simulink model "Bicycle_LKS"  (R2017a)
settings: Solver=ode45  StartTime=0.0  StopTime=20  FixedStep=1/120  MaxStep=1/120  RelTol=1e-3  EnableMultiTasking=on
InitFcn:
  | % Load matfile %
  | load('Matrix.mat')
  | load('PathData.mat')
  | 
  | % 차량의 초기 위치 및 속도 설정 %
  | X0 = 25;            % 초기 X좌표 [m]
  | Y0 = 0.00138;       % 초기 Y좌표 [m]
  | psi0 = -0.6*pi/180; % 초기 각도 [rad]
  | Vx0 = 100;          % 초기 속도 [km/h]
  | tf = 30;            % 시뮬레이션 시간 [s]
  | 
  | % % 제어기 설정 %
  | Q1 = 5;        % Lateral Offset 의 가중치
  | Q2 = 30;        % Drift Angle의 가중치
  | R =  250;       % Steering Angle의 가중치
  | PL = [-50-50i,-50+50i,-30,-20]; % Observer 극점
  | 
  | [K,L] = sfGain(Q1,Q2,R,PL);
model workspace (MAT data in the model file):
  Cf = 53220
  Cr = 39017
  Fy_Angle = [-20; -16; -14; -12; -10; -9.5; -9; -8.5; -8; -7.5; -7; -6.5; -6; -5.5; -5; -4.5; -4; -3.5; -3; -2.5; -2; -1.5; -1; -0.5; 0; 0.5; 1; 1.5; 2; 2.5; 3; 3.5; 4; 4.5; 5; 5.5; 6; 6.5; 7; 7.5; 8; 8.5; 9; 9.5; 10; 12; 14; 16; 18; 20]
  Fy_Data = [-1523.64 -1531.91 -1546.58 -1574.53 -1631.62 -1653.27 -1678.67 -1707.8 -1740.18 -1775.12 -1810.95 -1845.3 ... (250 elements, 50x5)]
  Fy_W = [1725 3500 6100 6950 9005]
  GearRatio = 17.25
  Izz = 4192
  P = [2.59634065709e-08 -1.77089434361e-05 0.0015503820009 -0.0564733379764 0.710785401626]
  lf = 1.11
  lr = 1.6662
  m = 1530
values from neighbouring files (symbols this model uses):
  K = lqr(A,B,Q,R)    [sfGain.m]
  L = place(A',C',PL)    [sfGain.m]
undefined symbols (not defined in the file or in its folder): A, B
libraries: simulink x1
settings Model: Creator=Park  LastModifiedBy=edward
settings DataIOCC: SaveFormat=Array  SignalLoggingSaveFormat=ModelDataLogs
settings OptimizationCC: ExpressionDepthLimit=2147483647  LifeSpan=inf
settings DebuggingCC: UnderspecifiedInitializationDetection=Classic  MergeDetectMultiDrivingBlocksExec=none  SolverPrmCheckMsg=warning  MultiTaskDSMMsg=warning  MultiTaskCondExecSysMsg=none  FcnCallInpInsideContextMsg=warning  StateNameClashWarn=warning  SFUnexpectedBacktrackingDiag=warning  SFNoUnconditionalDefaultTransitionDiag=warning  SFExecutionAtInitializationDiag=none
settings HardwareCC: ProdBitPerPointer=32  ProdBitPerSizeT=32  ProdBitPerPtrDiffT=32  ProdLargestAtomicFloat=None  ProdIntDivRoundTo=Undefined  ProdEndianess=Unspecified  ProdWordSize=32  ProdHWDeviceType=32-bit Generic
settings ModelReferenceCC: PropagateSignalLabelsOutOfModel=off
settings GRTTargetCC: TargetLangStandard=C89/C90 (ANSI)  GeneratePreprocessorConditionals=Disable all  CombineOutputUpdateFcns=off  GRTInterface=on
settings ConfigComp: CovMetricSettings=dw  CovHtmlReporting=on  CovSaveCumulativeToWorkspaceVar=on  CovSaveSingleToWorkspaceVar=on  CovExternalEMLEnable=off

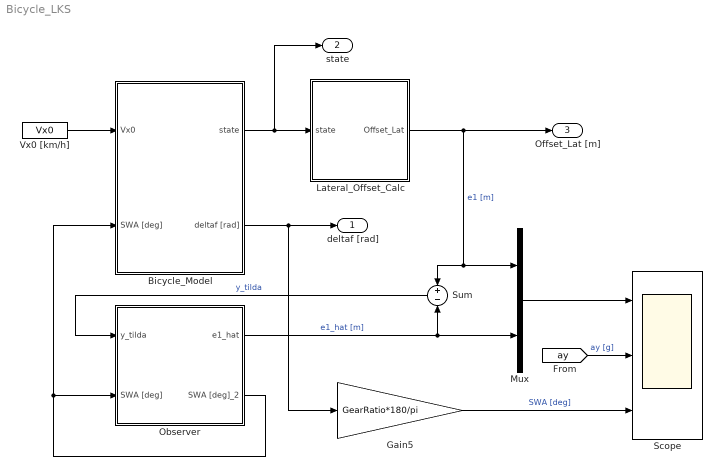
== system Bicycle_LKS ==
  Bicycle_Model : Subsystem
  Gain5 : Gain  Gain=GearRatio*180/pi
  Lateral_Offset_Calc : Subsystem  TreatAsAtomicUnit=on  SystemSampleTime=1/120
  Mux : Mux  Inputs=2
  Observer : Subsystem
  Scope : Scope  NumInputPorts=3
  Sum : Sum  Inputs=+-
  Vx0 [km/h] : Constant  Value=Vx0
  deltaf [rad] : Outport
  state : Outport  Port=2
  Offset_Lat [m] : Outport  Port=3
  wires:
  Bicycle_Model/1(state) -> Lateral_Offset_Calc/1(state), state/1
  Lateral_Offset_Calc/1(Offset_Lat) -> Offset_Lat [m]/1, Sum/1, Mux/1  "e1 [m]"
  Observer/1(e1_hat) -> Sum/2, Mux/2  "e1_hat [m]"
  Vx0 [km/h]/1 -> Bicycle_Model/1(Vx0)
  Sum/1 -> Observer/1(y_tilda)  "y_tilda"
  Mux/1 -> Scope/1
  [ay] -> Scope/2  "ay [g]"
  Bicycle_Model/2(deltaf [rad]) -> Gain5/1, deltaf [rad]/1
  Gain5/1 -> Scope/3  "SWA [deg]"
  Observer/2(SWA [deg]_2) -> Observer/2(SWA [deg]), Bicycle_Model/2(SWA [deg])

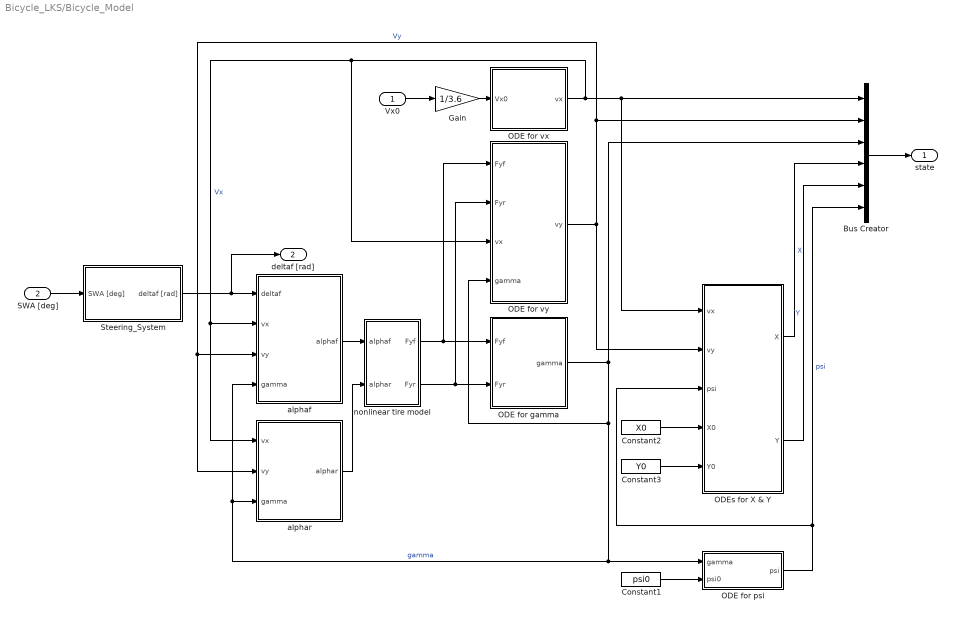
== system Bicycle_LKS/Bicycle_Model ==
  Vx0 : Inport
  SWA [deg] : Inport  Port=2
  Bus Creator : BusCreator  Inputs=6
  Constant1 : Constant  Value=psi0
  Constant2 : Constant  Value=X0
  Constant3 : Constant  Value=Y0
  Gain : Gain  Gain=1/3.6
  ODE for gamma : Subsystem
  ODE for psi : Subsystem
  ODE for vx : Subsystem
  ODE for vy : Subsystem
  ODEs for X & Y : Subsystem
  Steering_System : Subsystem
  alphaf : Subsystem
  alphar : Subsystem
  nonlinear tire model : Subsystem
  state : Outport
  deltaf [rad] : Outport  Port=2
  wires:
  alphaf/1(alphaf) -> nonlinear tire model/1(alphaf)
  alphar/1(alphar) -> nonlinear tire model/2(alphar)
  nonlinear tire model/1(Fyf) -> ODE for gamma/1(Fyf), ODE for vy/1(Fyf)
  nonlinear tire model/2(Fyr) -> ODE for gamma/2(Fyr), ODE for vy/2(Fyr)
  ODE for gamma/1(gamma) -> ODE for vy/4(gamma), alphar/3(gamma), alphaf/4(gamma), ODE for psi/1(gamma), Bus Creator/3  "gamma"
  ODE for vy/1(vy) -> Bus Creator/2, alphaf/3(vy), alphar/2(vy), ODEs for X & Y/2(vy)  "Vy"
  Bus Creator/1 -> state/1
  ODE for vx/1(vx) -> Bus Creator/1, ODEs for X & Y/1(vx), alphaf/2(vx), alphar/1(vx), ODE for vy/3(vx)  "Vx"
  Vx0/1 -> Gain/1
  Constant1/1 -> ODE for psi/2(psi0)
  Gain/1 -> ODE for vx/1(Vx0)
  SWA [deg]/1 -> Steering_System/1(SWA [deg])
  Steering_System/1(deltaf [rad]) -> deltaf [rad]/1, alphaf/1(deltaf)
  Constant2/1 -> ODEs for X & Y/4(X0)
  Constant3/1 -> ODEs for X & Y/5(Y0)
  ODE for psi/1(psi) -> Bus Creator/6, ODEs for X & Y/3(psi)  "psi"
  ODEs for X & Y/1(X) -> Bus Creator/4  "X"
  ODEs for X & Y/2(Y) -> Bus Creator/5  "Y"

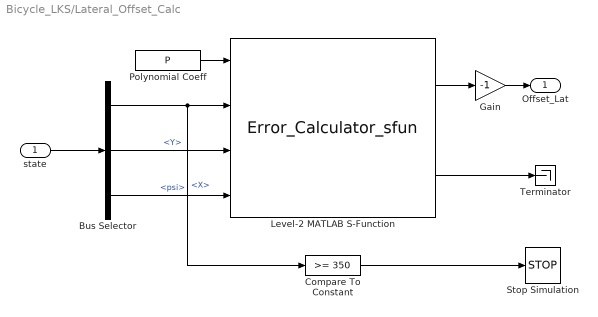
== system Bicycle_LKS/Lateral_Offset_Calc ==
  state : Inport
  Bus Selector : BusSelector  OutputSignals=X,Y,psi
  Compare To Constant : simulink/Logic and Bit Operations/Compare To Constant  relop=>=  const=350  OutDataTypeStr=boolean
  Gain : Gain  Gain=-1
  Level-2 MATLAB S-Function : M-S-Function  FunctionName=Error_Calculator_sfun
  Polynomial Coeff : Constant  Value=P
  Stop Simulation : Stop
  Terminator : Terminator
  Offset_Lat : Outport
  wires:
  state/1 -> Bus Selector/1
  Bus Selector/3 -> Level-2 MATLAB S-Function/4  "<psi>"
  Bus Selector/2 -> Level-2 MATLAB S-Function/3  "<Y>"
  Bus Selector/1 -> Compare To Constant/1, Level-2 MATLAB S-Function/2  "<X>"
  Level-2 MATLAB S-Function/1 -> Gain/1
  Polynomial Coeff/1 -> Level-2 MATLAB S-Function/1
  Level-2 MATLAB S-Function/2 -> Terminator/1
  Gain/1 -> Offset_Lat/1
  Compare To Constant/1 -> Stop Simulation/1

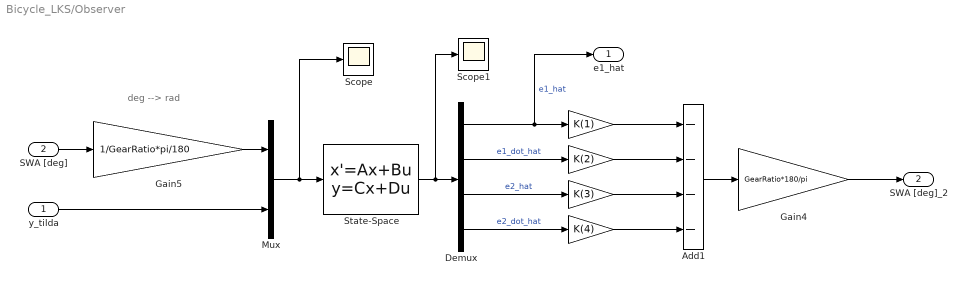
== system Bicycle_LKS/Observer ==
  note: deg --> rad
  y_tilda : Inport
  SWA [deg] : Inport  Port=2
  " " : Gain  Gain=K(1)
  "  " : Gain  Gain=K(2)
  "   " : Gain  Gain=K(3)
  "    " : Gain  Gain=K(4)
  Add1 : Sum  Inputs=----
  Demux : Demux
  Gain4 : Gain  Gain=GearRatio*180/pi
  Gain5 : Gain  Gain=1/GearRatio*pi/180
  Mux : Mux  Inputs=2
  Scope : Scope
  Scope1 : Scope
  State-Space : StateSpace  A=A  B=[B L']  C=diag([1 1 1 1])  D=zeros(4,2)  X0=0  ContinuousStateAttributes={'e1','e1_dot','e2','e2_dot'}
  e1_hat : Outport
  SWA [deg]_2 : Outport  Port=2
  wires:
  Mux/1 -> State-Space/1, Scope/1
  State-Space/1 -> Scope1/1, Demux/1
  Demux/1 -> e1_hat/1, " "/1  "e1_hat"
  y_tilda/1 -> Mux/2
  Demux/3 -> "   "/1  "e2_hat"
  Demux/2 -> "  "/1  "e1_dot_hat"
  Demux/4 -> "    "/1  "e2_dot_hat"
  SWA [deg]/1 -> Gain5/1
  Gain5/1 -> Mux/1
  "    "/1 -> Add1/4
  "   "/1 -> Add1/3
  "  "/1 -> Add1/2
  " "/1 -> Add1/1
  Add1/1 -> Gain4/1
  Gain4/1 -> SWA [deg]_2/1

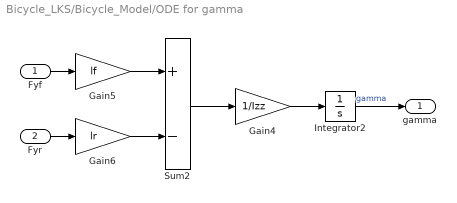
== system Bicycle_LKS/Bicycle_Model/ODE for gamma ==
  Fyf : Inport
  Fyr : Inport  Port=2
  Gain4 : Gain  Gain=1/Izz
  Gain5 : Gain  Gain=lf
  Gain6 : Gain  Gain=lr
  Integrator2 : Integrator
  Sum2 : Sum  Inputs=+-
  gamma : Outport
  wires:
  Sum2/1 -> Gain4/1
  Gain4/1 -> Integrator2/1
  Gain5/1 -> Sum2/1
  Gain6/1 -> Sum2/2
  Fyf/1 -> Gain5/1
  Integrator2/1 -> gamma/1  "gamma"
  Fyr/1 -> Gain6/1

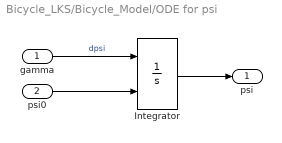
== system Bicycle_LKS/Bicycle_Model/ODE for psi ==
  gamma : Inport
  psi0 : Inport  Port=2
  Integrator : Integrator  InitialConditionSource=external
  psi : Outport
  wires:
  gamma/1 -> Integrator/1  "dpsi"
  Integrator/1 -> psi/1
  psi0/1 -> Integrator/2

== system Bicycle_LKS/Bicycle_Model/ODE for vx ==
  Vx0 : Inport
  Constant : Constant  Value=0
  Integrator1 : Integrator  InitialConditionSource=external  InitialCondition=80/3.6
  vx : Outport
  wires:
  Constant/1 -> Integrator1/1  "dvx"
  Integrator1/1 -> vx/1  "vx"
  Vx0/1 -> Integrator1/2

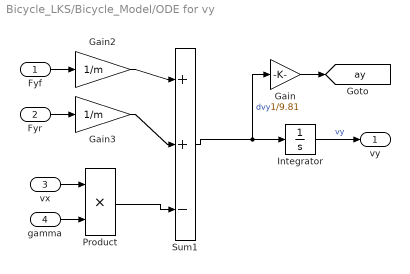
== system Bicycle_LKS/Bicycle_Model/ODE for vy ==
  Fyf : Inport
  Fyr : Inport  Port=2
  vx : Inport  Port=3
  gamma : Inport  Port=4
  Gain : Gain  Gain=1/9.81
  Gain2 : Gain  Gain=1/m
  Gain3 : Gain  Gain=1/m
  Integrator : Integrator
  Product : Product  RndMeth=Zero
  Sum1 : Sum  Inputs=++|-
  vy : Outport
  tag scope: ay=global
  wires:
  Gain2/1 -> Sum1/1
  Gain3/1 -> Sum1/2
  Sum1/1 -> Gain/1, Integrator/1  "dvy"
  Product/1 -> Sum1/3
  Fyf/1 -> Gain2/1
  Fyr/1 -> Gain3/1
  Integrator/1 -> vy/1  "vy"
  vx/1 -> Product/1
  gamma/1 -> Product/2
  Gain/1 -> [ay]

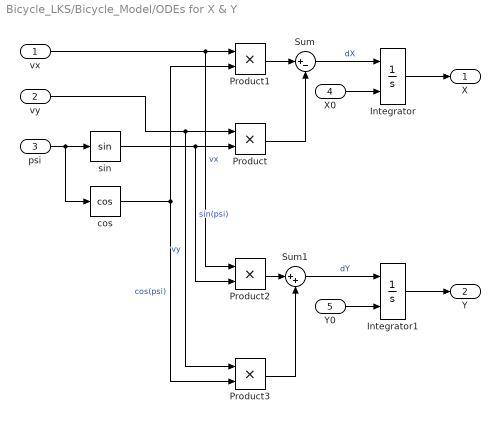
== system Bicycle_LKS/Bicycle_Model/ODEs for X & Y ==
  vx : Inport
  vy : Inport  Port=2
  psi : Inport  Port=3
  X0 : Inport  Port=4
  Y0 : Inport  Port=5
  Integrator : Integrator  InitialConditionSource=external  InitialCondition=42.14
  Integrator1 : Integrator  InitialConditionSource=external  InitialCondition=-0.3743
  Product{,1..3} (4 alike) : Product  RndMeth=Zero
  Sum : Sum  Inputs=|+-
  Sum1 : Sum  Inputs=|++
  cos : Trigonometry  Operator=cos
  sin : Trigonometry
  X : Outport
  Y : Outport  Port=2
  wires:
  psi/1 -> sin/1, cos/1
  sin/1 -> Product/2, Product2/2  "sin(psi)"
  vy/1 -> Product/1, Product3/1  "vy"
  vx/1 -> Product1/1, Product2/1  "vx"
  cos/1 -> Product1/2, Product3/2  "cos(psi)"
  Product1/1 -> Sum/1
  Product/1 -> Sum/2
  Sum/1 -> Integrator/1  "dX"
  Product2/1 -> Sum1/1
  Product3/1 -> Sum1/2
  Sum1/1 -> Integrator1/1  "dY"
  Integrator/1 -> X/1
  Integrator1/1 -> Y/1
  X0/1 -> Integrator/2
  Y0/1 -> Integrator1/2

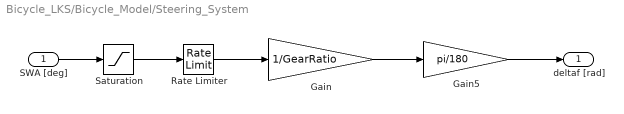
== system Bicycle_LKS/Bicycle_Model/Steering_System ==
  SWA [deg] : Inport
  Gain : Gain  Gain=1/GearRatio
  Gain5 : Gain  Gain=pi/180
  Rate Limiter : RateLimiter  RisingSlewLimit=500  FallingSlewLimit=-500  SampleTimeMode=inherited
  Saturation : Saturate  UpperLimit=450  LowerLimit=-450
  deltaf [rad] : Outport
  wires:
  Gain/1 -> Gain5/1
  Gain5/1 -> deltaf [rad]/1
  SWA [deg]/1 -> Saturation/1
  Rate Limiter/1 -> Gain/1
  Saturation/1 -> Rate Limiter/1

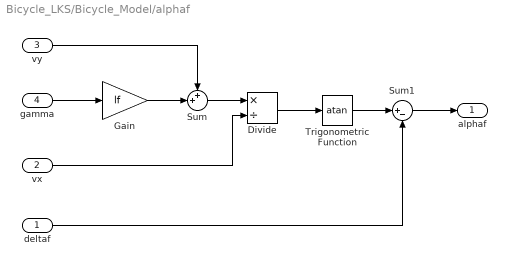
== system Bicycle_LKS/Bicycle_Model/alphaf ==
  deltaf : Inport
  vx : Inport  Port=2
  vy : Inport  Port=3
  gamma : Inport  Port=4
  Divide : Product  Inputs=*/
  Gain : Gain  Gain=lf
  Sum : Sum  Inputs=++|
  Sum1 : Sum  Inputs=|+-
  Trigonometric Function : Trigonometry  Operator=atan
  alphaf : Outport
  wires:
  gamma/1 -> Gain/1
  vy/1 -> Sum/1
  Gain/1 -> Sum/2
  Sum/1 -> Divide/1
  vx/1 -> Divide/2
  Divide/1 -> Trigonometric Function/1
  Trigonometric Function/1 -> Sum1/1
  deltaf/1 -> Sum1/2
  Sum1/1 -> alphaf/1

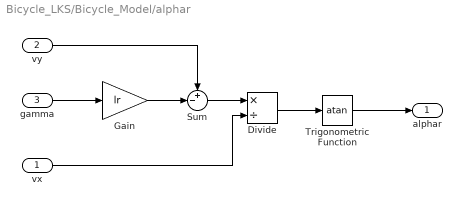
== system Bicycle_LKS/Bicycle_Model/alphar ==
  vx : Inport
  vy : Inport  Port=2
  gamma : Inport  Port=3
  Divide : Product  Inputs=*/
  Gain : Gain  Gain=lr
  Sum : Sum  Inputs=+-|
  Trigonometric Function : Trigonometry  Operator=atan
  alphar : Outport
  wires:
  Trigonometric Function/1 -> alphar/1
  Divide/1 -> Trigonometric Function/1
  vx/1 -> Divide/2
  Sum/1 -> Divide/1
  Gain/1 -> Sum/2
  vy/1 -> Sum/1
  gamma/1 -> Gain/1

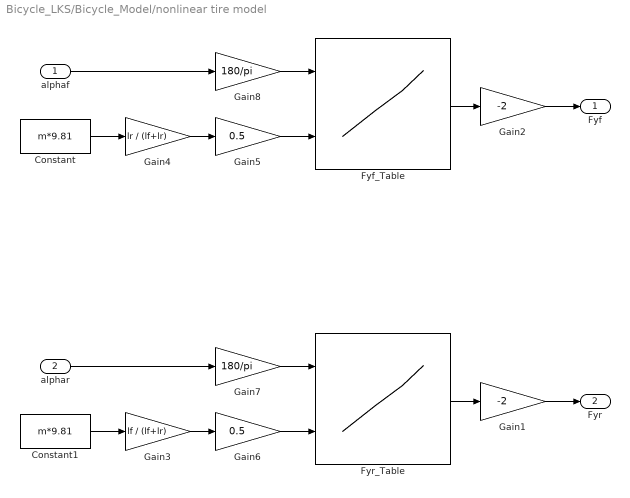
== system Bicycle_LKS/Bicycle_Model/nonlinear tire model ==
  alphaf : Inport
  alphar : Inport  Port=2
  Constant : Constant  Value=m*9.81
  Constant1 : Constant  Value=m*9.81
  Fyf_Table : Lookup2D  RowIndex=Fy_Angle  ColumnIndex=Fy_W  Table=Fy_Data  LookUpMeth=Interpolation-Use End Values  SaturateOnIntegerOverflow=on
  Fyr_Table : Lookup2D  RowIndex=Fy_Angle  ColumnIndex=Fy_W  Table=Fy_Data  LookUpMeth=Interpolation-Use End Values  SaturateOnIntegerOverflow=on
  Gain1 : Gain  Gain=-2
  Gain2 : Gain  Gain=-2
  Gain3 : Gain  Gain=lf / (lf+lr)
  Gain4 : Gain  Gain=lr / (lf+lr)
  Gain5 : Gain  Gain=0.5
  Gain6 : Gain  Gain=0.5
  Gain7 : Gain  Gain=180/pi
  Gain8 : Gain  Gain=180/pi
  Fyf : Outport
  Fyr : Outport  Port=2
  wires:
  alphaf/1 -> Gain8/1
  Constant/1 -> Gain4/1
  Gain4/1 -> Gain5/1
  Gain5/1 -> Fyf_Table/2
  Fyf_Table/1 -> Gain2/1
  Gain2/1 -> Fyf/1
  Gain8/1 -> Fyf_Table/1
  alphar/1 -> Gain7/1
  Gain3/1 -> Gain6/1
  Gain6/1 -> Fyr_Table/2
  Fyr_Table/1 -> Gain1/1
  Gain7/1 -> Fyr_Table/1
  Constant1/1 -> Gain3/1
  Gain1/1 -> Fyr/1
